simulink model "ingaszabsim"  (R2013a)
settings: Solver=ode45  StartTime=0.0  StopTime=60  RelTol=1e-3
values from neighbouring files (symbols this model uses):
  b = 100    [Ingaszab.m]
  fi0 = 10/180*pi    (= 0.174532925199)    [Ingaszab.m]
  g = 9.81    [Ingaszab.m]
  J = 0.008    [Ingaszab.m]
  l = 0.14    [Ingaszab.m]
  m = 0.4    [Ingaszab.m]
  M = 0.6    [Ingaszab.m]
  x0 = 5    [Ingaszab.m]
libraries: simulink x1
settings Model: Creator=Kinga  LastModifiedBy=rudi
settings DataIOCC: SignalLoggingSaveFormat=ModelDataLogs
settings DebuggingCC: UnderspecifiedInitializationDetection=Simplified  MultiTaskDSMMsg=warning  MultiTaskCondExecSysMsg=none  StateNameClashWarn=none  StrictBusMsg=ErrorOnBusTreatedAsVector  NonBusSignalsTreatedAsBus=error
settings RTWCC: IncludeERTFirstTime=on
settings GRTTargetCC: CodeReplacementLibrary=None  CPPClassGenCompliant=on

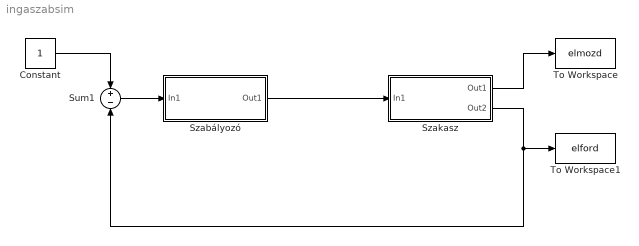
== system ingaszabsim ==
  Constant : Constant
  Sum1 : Sum  Inputs=+-
  Szabályozó : Subsystem
  Szakasz : Subsystem
  To Workspace : ToWorkspace  VariableName=elmozd  SampleTime=-1  SaveFormat=Timeseries
  To Workspace1 : ToWorkspace  VariableName=elford  SampleTime=-1  SaveFormat=Timeseries
  wires:
  Szabályozó/1(Out1) -> Szakasz/1(In1)
  Szakasz/1(Out1) -> To Workspace/1
  Szakasz/2(Out2) -> To Workspace1/1, Sum1/2
  Sum1/1 -> Szabályozó/1(In1)
  Constant/1 -> Sum1/1

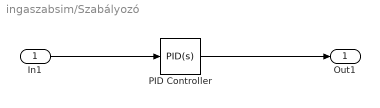
== system ingaszabsim/Szabályozó ==
  In1 : Inport
  PID Controller : simulink/Continuous/PID Controller  Controller=PID  TimeDomain=Continuous-time  SampleTime=1  IntegratorMethod=Forward Euler  FilterMethod=Forward Euler  Form=Parallel  P=-56638.6052262267  I=-2674171.19181056  D=-281.297389048913  N=1854.51647807346  InitialConditionSource=internal  InitialConditionForIntegrator=0  InitialConditionForFilter=0  ExternalReset=none  LimitOutput=off  UpperSaturationLimit=inf  LowerSaturationLimit=-inf  LinearizeAsGain=on  AntiWindupMode=none  Kb=1  TrackingMode=off  Kt=1  PParamMin=[]  PParamMax=[]  IParamMin=[]  IParamMax=[]  DParamMin=[]  DParamMax=[]  NParamMin=[]  NParamMax=[]  KbParamMin=[]  KbParamMax=[]  KtParamMin=[]  KtParamMax=[]  POutMin=[]  POutMax=[]  IOutMin=[]  IOutMax=[]  DOutMin=[]  DOutMax=[]  NOutMin=[]  NOutMax=[]  KbOutMin=[]  KbOutMax=[]  KtOutMin=[]  KtOutMax=[]  IntegratorOutMin=[]  IntegratorOutMax=[]  FilterOutMin=[]  FilterOutMax=[]  SumOutMin=[]  SumOutMax=[]  SumI1OutMin=[]  SumI1OutMax=[]  SumI2OutMin=[]  SumI2OutMax=[]  SumI3OutMin=[]  SumI3OutMax=[]  SumDOutMin=[]  SumDOutMax=[]  SaturationOutMin=[]  SaturationOutMax=[]  IntegratorContinuousStateAttributes=''  IntegratorStateMustResolveToSignalObject=off  IntegratorRTWStateStorageClass=Auto  FilterContinuousStateAttributes=''  FilterStateMustResolveToSignalObject=off  FilterRTWStateStorageClass=Auto
  Out1 : Outport
  wires:
  In1/1 -> PID Controller/1
  PID Controller/1 -> Out1/1

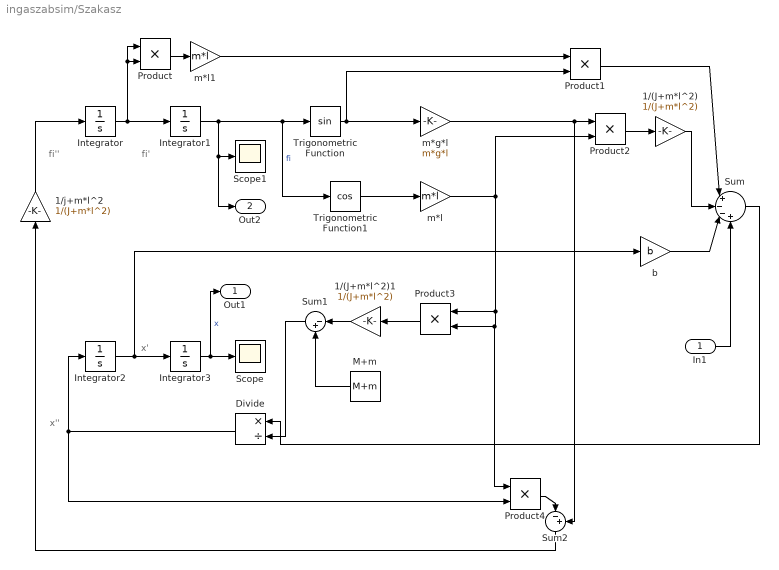
== system ingaszabsim/Szakasz ==
  note: x''
  note: x'
  note: fi''
  note: fi'
  In1 : Inport
  1/(J+m*l^2) : Gain  Gain=1/(J+m*l^2)
  1/(J+m*l^2)1 : Gain  Gain=1/(J+m*l^2)
  1/j+m*l^2 : Gain  Gain=1/(J+m*l^2)
  Divide : Product  Inputs=*/
  Integrator : Integrator
  Integrator1 : Integrator  InitialCondition=fi0
  Integrator2 : Integrator
  Integrator3 : Integrator  InitialCondition=x0
  M+m : Constant  Value=M+m
  Product{,1..4} (5 alike) : Product
  Scope : Scope
      settings: SaveName=ScopeData2
  Scope1 : Scope
      settings: TimeRange=30  YMin=0.016580635  YMax=0.018325965  SaveName=ScopeData3
  Sum : Sum  Inputs=|+--+
  Sum1 : Sum  Inputs=|-+
  Sum2 : Sum  Inputs=|-+
  Trigonometric Function : Trigonometry
  Trigonometric Function1 : Trigonometry  Operator=cos
  b : Gain  Gain=b
  m*g*l : Gain  Gain=m*g*l
  m*l : Gain  Gain=m*l
  m*l1 : Gain  Gain=m*l
  Out1 : Outport
  Out2 : Outport  Port=2
  wires:
  Integrator/1 -> Integrator1/1, Product/1, Product/2
  Integrator2/1 -> b/1, Integrator3/1
  Integrator1/1 -> Trigonometric Function1/1, Trigonometric Function/1, Out2/1, Scope1/1  "fi"
  Trigonometric Function/1 -> Product1/2, m*g*l/1
  Trigonometric Function1/1 -> m*l/1
  Product/1 -> m*l1/1
  m*l1/1 -> Product1/1
  m*g*l/1 -> Sum2/2, Product2/1
  m*l/1 -> Product3/1, Product3/2, Product4/1, Product2/2
  Product2/1 -> 1/(J+m*l^2)/1
  Product1/1 -> Sum/1
  1/(J+m*l^2)/1 -> Sum/2
  b/1 -> Sum/3
  Product3/1 -> 1/(J+m*l^2)1/1
  1/(J+m*l^2)1/1 -> Sum1/1
  Divide/1 -> Product4/2, Integrator2/1
  1/j+m*l^2/1 -> Integrator/1
  Product4/1 -> Sum2/1
  Sum2/1 -> 1/j+m*l^2/1
  Integrator3/1 -> Out1/1, Scope/1  "x"
  Sum1/1 -> Divide/2
  Sum/1 -> Divide/1
  In1/1 -> Sum/4
  M+m/1 -> Sum1/2
